simulink model "QUESTION3_2_CCF"  (R2021a)
settings: Solver=VariableStepAuto  StartTime=0.0  StopTime=10.0  RelTol=1e-3
settings Model: Creator=user  LastModifiedBy=user

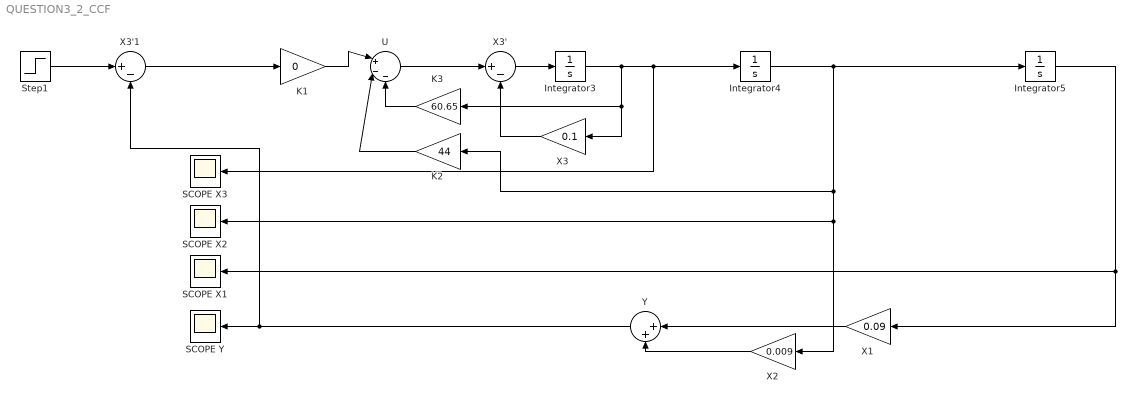
== system QUESTION3_2_CCF ==
  Integrator3 : Integrator
  Integrator4 : Integrator
  Integrator5 : Integrator
  K1 : Gain  Gain=0
  K2 : Gain  Gain=44
  K3 : Gain  Gain=60.65
  SCOPE X1 : Scope
  SCOPE X2 : Scope
  SCOPE X3 : Scope
  SCOPE Y : Scope
  Step1 : Step  SampleTime=0
  U : Sum  Inputs=|+--
  X1 : Gain  Gain=0.09
  X2 : Gain  Gain=0.009
  X3 : Gain  Gain=0.1
  X3' : Sum  Inputs=|+-
  X3'1 : Sum  Inputs=|+-
  Y : Sum  Inputs=|++
  wires:
  X3'/1 -> Integrator3/1
  Integrator3/1 -> SCOPE X3/1, Integrator4/1, K3/1, X3/1
  Integrator4/1 -> X2/1, SCOPE X2/1, K2/1, Integrator5/1
  X3/1 -> X3'/2
  Integrator5/1 -> X1/1, SCOPE X1/1
  X2/1 -> Y/2
  X1/1 -> Y/1
  Y/1 -> X3'1/2, SCOPE Y/1
  Step1/1 -> X3'1/1
  X3'1/1 -> K1/1
  K1/1 -> U/1
  U/1 -> X3'/1
  K3/1 -> U/3
  K2/1 -> U/2
